simulink model "cascademodel"  (R2023a)
settings: Solver=VariableStepAuto  StartTime=0.0  StopTime=1  FixedStep=0.03  RelTol=1e-3
values from neighbouring files (symbols this model uses):
  b_1 = 51.0314    [modelsetup.m]
  b_2 = -13.8341    [modelsetup.m]
  EPSILON = 0.005    [modelsetup.m]
  F_kinetic = 8.1003    [modelsetup.m]
  F_static = 10.4160    (= 10.416)    [modelsetup.m]
  J = 9.1617    [modelsetup.m]
  K = K_t / estimated_b    (= 0.904771025438)    [modelsetup.m]
  K_t = 0.124 * 120    (= 14.88)    [modelsetup.m]
  tau = J / estimated_b    (= 0.55707262794)    [modelsetup.m]
libraries: slpidlib x5
settings Model: Creator=yunzh  LastModifiedBy=yunzh

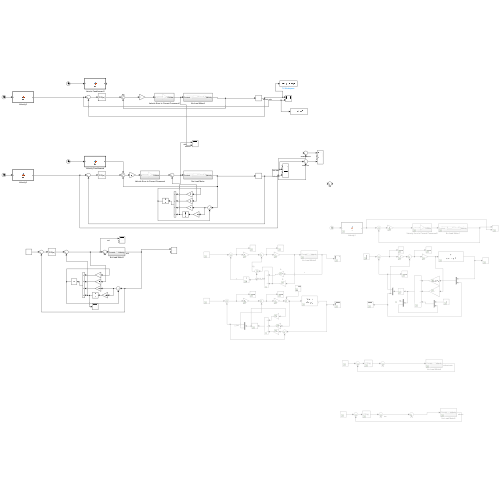
[thumbnail: Simulink's stored preview of the top-level diagram]
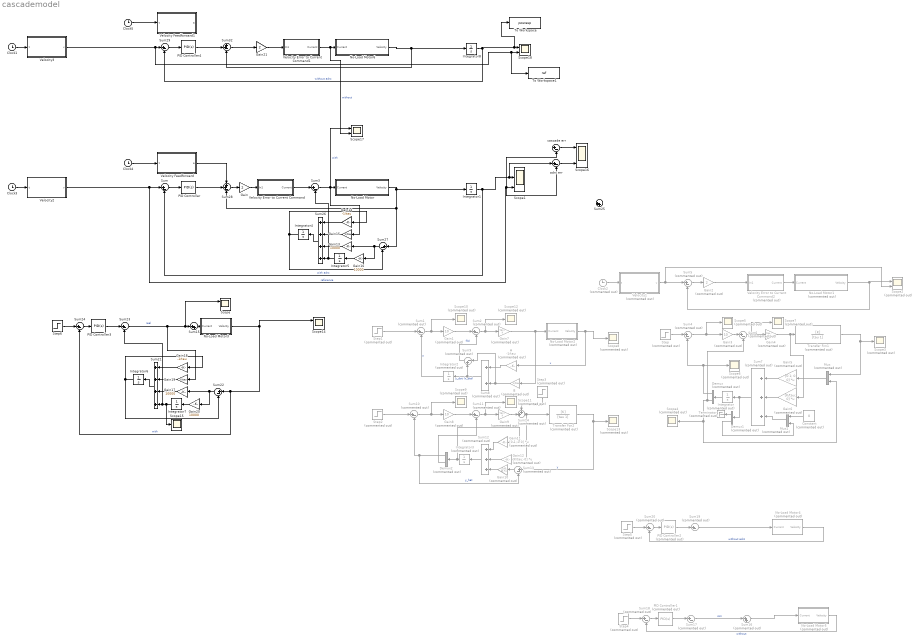
== system cascademodel ==
  A : Gain  Commented=on  Gain=-1/tau
  B : Gain  Commented=on  Gain=K/tau
  Clock{1,3..5} (4 alike) : Clock
  Clock2 : Clock  Commented=on
  Constant : Constant  Commented=on  Value=0
  Demux : Demux  Commented=on  Outputs=2
  Demux1 : Demux  Commented=on  Outputs=2
  Demux2 : Demux  Commented=on  Outputs=2
  Gain : Gain  Gain=2
  Gain1 : Gain  Commented=on  Gain=10
  Gain10 : Gain  Commented=on  Gain=[100; 0]  Multiplication=Matrix(K*u)
  Gain11 : Gain  Commented=on  Gain=[0 1; 0 0]  Multiplication=Matrix(K*u)
  Gain12 : Gain  Commented=on  Gain=[K/tau; 0]  Multiplication=Matrix(K*u)
  Gain{13,16..17,20} (4 alike) : Gain  Gain=10000
  Gain14 : Gain  Gain=-1\tau
  Gain15 : Gain  Gain=K/tau
  Gain18 : Gain  Gain=-1/tau
  Gain19 : Gain  Gain=K/tau
  Gain2 : Gain  Commented=on  Gain=2
  Gain21 : Gain  Gain=2
  Gain3 : Gain  Commented=on  Gain=10
  Gain4 : Gain  Commented=on  Gain=tau / K
  Gain5 : Gain  Commented=on  Gain=[0 1; 0 0]  Multiplication=Matrix(K*u)
  Gain6 : Gain  Commented=on  Gain=[K/tau; 0]  Multiplication=Matrix(K*u)
  Gain7 : Gain  Commented=on  Gain=tau / K
  Gain8 : Gain  Commented=on  Gain=10
  Gain9 : Gain  Commented=on  Gain=tau / K
  Integrator : Integrator  Commented=on
  Integrator{1,4..8} (6 alike) : Integrator
  Integrator2 : Integrator  Commented=on
  Integrator3 : Integrator  Commented=on
  Mux : Mux  Commented=on  Inputs=2
  Mux1 : Mux  Commented=on  Inputs=2
  No-Load Motor : Subsystem
  No-Load Motor1 : Subsystem  Commented=on
  No-Load Motor2 : Subsystem  Commented=on
  No-Load Motor3 : Subsystem
  No-Load Motor4 : Subsystem  Commented=on
  No-Load Motor5 : Subsystem  Commented=on
  No-Load Motor6 : Subsystem
  PID Controller : slpidlib/PID Controller  Controller=PID  Form=Parallel  TimeDomain=Continuous-time  UseExternalTs=off  SampleTime=-1  IntegratorMethod=Forward Euler  FilterMethod=Forward Euler  ControllerParametersSource=internal  P=10  I=1  UseKiTs=off  D=0  N=100  UseFilter=on  TunerSelectOption=Transfer Function Based (PID Tuner App)  InitialConditionSource=internal  InitialConditionForIntegrator=0  InitialConditionForFilter=0  DifferentiatorICPrevScaledInput=0  ExternalReset=none  TrackingMode=off  Kt=1  LimitOutput=off  SatLimitsSource=internal  UpperSaturationLimit=inf  LowerSaturationLimit=-inf  LinearizeAsGain=on  AntiWindupMode=none  Kb=1  LimitIntegrator=off  UpperIntegratorSaturationLimit=inf  LowerIntegratorSaturationLimit=-inf  POutMin=[]  POutMax=[]  IOutMin=[]  IOutMax=[]  DOutMin=[]  DOutMax=[]  NOutMin=[]  NOutMax=[]  SumOutMin=[]  SumOutMax=[]  SaturationOutMin=[]  SaturationOutMax=[]  PParamMin=[]  PParamMax=[]  IParamMin=[]  IParamMax=[]  DParamMin=[]  DParamMax=[]  NParamMin=[]  NParamMax=[]  KbParamMin=[]  KbParamMax=[]  KtParamMin=[]  KtParamMax=[]  KbOutMin=[]  KbOutMax=[]  KtOutMin=[]  KtOutMax=[]  IntegratorOutMin=[]  IntegratorOutMax=[]  FilterOutMin=[]  FilterOutMax=[]  SumI1OutMin=[]  SumI1OutMax=[]  SumI2OutMin=[]  SumI2OutMax=[]  SumI3OutMin=[]  SumI3OutMax=[]  SumI4OutMin=[]  SumI4OutMax=[]  SumDOutMin=[]  SumDOutMax=[]  DifferentiatorOutMin=[]  DifferentiatorOutMax=[]  FilterDiffOutCoefMin=[]  FilterDiffOutCoefMax=[]  ReciprocalOutMin=[]  ReciprocalOutMax=[]  SumDenOutMin=[]  SumDenOutMax=[]  SumNumOutMin=[]  SumNumOutMax=[]  DivideOutMin=[]  DivideOutMax=[]  UdiffTsProdOutMin=[]  UdiffTsProdOutMax=[]  NTsProdOutMin=[]  NTsProdOutMax=[]  UintegralTsProdOutMin=[]  UintegralTsProdOutMax=[]  UngainTsProdOutMin=[]  UngainTsProdOutMax=[]  ClampingZeroOutDataTypeStr=Inherit: Inherit via back propagation  ClampingZeroOutMin=[]  ClampingZeroOutMax=[]  FilterDenConstantOutDataTypeStr=Inherit: Inherit via back propagation  FilterDenConstantOutMin=[]  FilterDenConstantOutMax=[]  PCopyOutDataTypeStr=Inherit: Inherit via back propagation  PCopyOutMin=[]  PCopyOutMax=[]  NCopyOutDataTypeStr=Inherit: Inherit via back propagation  NCopyOutMin=[]  NCopyOutMax=[]  IntegratorContinuousStateAttributes=''  IntegratorStateMustResolveToSignalObject=off  IntegratorRTWStateStorageClass=Auto  FilterContinuousStateAttributes=''  FilterStateMustResolveToSignalObject=off  FilterRTWStateStorageClass=Auto  ParallelPVariant=InternalParameters  IdealPVariant=Disabled  IVariant=InternalParameters  DVariant=InternalParameters  IntegratorVariant=Continuous  SatVariant=Disabled  AWVariant=Passthrough  PCopyVariant=Disabled  TRVariant=Disabled  FdbkBlocksVariant=Forward  IdealPFdbkVariant=Disabled  SatFdbkVariant=Disabled  DerivativeFilterVariant=ContFilter  NVariant=InternalParameters  NCopyVariant=Disabled  FilterICVariant=InternalICsFilter  IntegratorICVariant=InternalICs  ExternalResetVariant=Disabled  TRSumVariant=Passthrough  SumFdbkVariant=Disabled  SumVariant=Sum_PID  TsampFilterVariant=InternalTs  TsampNgainVariant=Passthrough  TsampIntegralVariant=Disabled_SignalSpec  ExternalSaturationOutDataTypeStr=Inherit: Same as second input
  PID Controller1 : slpidlib/PID Controller  Commented=on  Controller=PID  Form=Parallel  TimeDomain=Continuous-time  UseExternalTs=off  SampleTime=-1  IntegratorMethod=Forward Euler  FilterMethod=Forward Euler  ControllerParametersSource=internal  P=5  I=1  UseKiTs=off  D=0  N=100  UseFilter=on  TunerSelectOption=Transfer Function Based (PID Tuner App)  InitialConditionSource=internal  InitialConditionForIntegrator=0  InitialConditionForFilter=0  DifferentiatorICPrevScaledInput=0  ExternalReset=none  TrackingMode=off  Kt=1  LimitOutput=off  SatLimitsSource=internal  UpperSaturationLimit=inf  LowerSaturationLimit=-inf  LinearizeAsGain=on  AntiWindupMode=none  Kb=1  LimitIntegrator=off  UpperIntegratorSaturationLimit=inf  LowerIntegratorSaturationLimit=-inf  POutMin=[]  POutMax=[]  IOutMin=[]  IOutMax=[]  DOutMin=[]  DOutMax=[]  NOutMin=[]  NOutMax=[]  SumOutMin=[]  SumOutMax=[]  SaturationOutMin=[]  SaturationOutMax=[]  PParamMin=[]  PParamMax=[]  IParamMin=[]  IParamMax=[]  DParamMin=[]  DParamMax=[]  NParamMin=[]  NParamMax=[]  KbParamMin=[]  KbParamMax=[]  KtParamMin=[]  KtParamMax=[]  KbOutMin=[]  KbOutMax=[]  KtOutMin=[]  KtOutMax=[]  IntegratorOutMin=[]  IntegratorOutMax=[]  FilterOutMin=[]  FilterOutMax=[]  SumI1OutMin=[]  SumI1OutMax=[]  SumI2OutMin=[]  SumI2OutMax=[]  SumI3OutMin=[]  SumI3OutMax=[]  SumI4OutMin=[]  SumI4OutMax=[]  SumDOutMin=[]  SumDOutMax=[]  DifferentiatorOutMin=[]  DifferentiatorOutMax=[]  FilterDiffOutCoefMin=[]  FilterDiffOutCoefMax=[]  ReciprocalOutMin=[]  ReciprocalOutMax=[]  SumDenOutMin=[]  SumDenOutMax=[]  SumNumOutMin=[]  SumNumOutMax=[]  DivideOutMin=[]  DivideOutMax=[]  UdiffTsProdOutMin=[]  UdiffTsProdOutMax=[]  NTsProdOutMin=[]  NTsProdOutMax=[]  UintegralTsProdOutMin=[]  UintegralTsProdOutMax=[]  UngainTsProdOutMin=[]  UngainTsProdOutMax=[]  ClampingZeroOutDataTypeStr=Inherit: Inherit via back propagation  ClampingZeroOutMin=[]  ClampingZeroOutMax=[]  FilterDenConstantOutDataTypeStr=Inherit: Inherit via back propagation  FilterDenConstantOutMin=[]  FilterDenConstantOutMax=[]  PCopyOutDataTypeStr=Inherit: Inherit via back propagation  PCopyOutMin=[]  PCopyOutMax=[]  NCopyOutDataTypeStr=Inherit: Inherit via back propagation  NCopyOutMin=[]  NCopyOutMax=[]  IntegratorContinuousStateAttributes=''  IntegratorStateMustResolveToSignalObject=off  IntegratorRTWStateStorageClass=Auto  FilterContinuousStateAttributes=''  FilterStateMustResolveToSignalObject=off  FilterRTWStateStorageClass=Auto  ParallelPVariant=InternalParameters  IdealPVariant=Disabled  IVariant=InternalParameters  DVariant=InternalParameters  IntegratorVariant=Continuous  SatVariant=Disabled  AWVariant=Passthrough  PCopyVariant=Disabled  TRVariant=Disabled  FdbkBlocksVariant=Forward  IdealPFdbkVariant=Disabled  SatFdbkVariant=Disabled  DerivativeFilterVariant=ContFilter  NVariant=InternalParameters  NCopyVariant=Disabled  FilterICVariant=InternalICsFilter  IntegratorICVariant=InternalICs  ExternalResetVariant=Disabled  TRSumVariant=Passthrough  SumFdbkVariant=Disabled  SumVariant=Sum_PID  TsampFilterVariant=InternalTs  TsampNgainVariant=Passthrough  TsampIntegralVariant=Disabled_SignalSpec  ExternalSaturationOutDataTypeStr=Inherit: Same as second input
  PID Controller2 : slpidlib/PID Controller  Commented=on  Controller=PID  Form=Parallel  TimeDomain=Continuous-time  UseExternalTs=off  SampleTime=-1  IntegratorMethod=Forward Euler  FilterMethod=Forward Euler  ControllerParametersSource=internal  P=1  I=1  UseKiTs=off  D=0  N=100  UseFilter=on  TunerSelectOption=Transfer Function Based (PID Tuner App)  InitialConditionSource=internal  InitialConditionForIntegrator=0  InitialConditionForFilter=0  DifferentiatorICPrevScaledInput=0  ExternalReset=none  TrackingMode=off  Kt=1  LimitOutput=off  SatLimitsSource=internal  UpperSaturationLimit=inf  LowerSaturationLimit=-inf  LinearizeAsGain=on  AntiWindupMode=none  Kb=1  LimitIntegrator=off  UpperIntegratorSaturationLimit=inf  LowerIntegratorSaturationLimit=-inf  POutMin=[]  POutMax=[]  IOutMin=[]  IOutMax=[]  DOutMin=[]  DOutMax=[]  NOutMin=[]  NOutMax=[]  SumOutMin=[]  SumOutMax=[]  SaturationOutMin=[]  SaturationOutMax=[]  PParamMin=[]  PParamMax=[]  IParamMin=[]  IParamMax=[]  DParamMin=[]  DParamMax=[]  NParamMin=[]  NParamMax=[]  KbParamMin=[]  KbParamMax=[]  KtParamMin=[]  KtParamMax=[]  KbOutMin=[]  KbOutMax=[]  KtOutMin=[]  KtOutMax=[]  IntegratorOutMin=[]  IntegratorOutMax=[]  FilterOutMin=[]  FilterOutMax=[]  SumI1OutMin=[]  SumI1OutMax=[]  SumI2OutMin=[]  SumI2OutMax=[]  SumI3OutMin=[]  SumI3OutMax=[]  SumI4OutMin=[]  SumI4OutMax=[]  SumDOutMin=[]  SumDOutMax=[]  DifferentiatorOutMin=[]  DifferentiatorOutMax=[]  FilterDiffOutCoefMin=[]  FilterDiffOutCoefMax=[]  ReciprocalOutMin=[]  ReciprocalOutMax=[]  SumDenOutMin=[]  SumDenOutMax=[]  SumNumOutMin=[]  SumNumOutMax=[]  DivideOutMin=[]  DivideOutMax=[]  UdiffTsProdOutMin=[]  UdiffTsProdOutMax=[]  NTsProdOutMin=[]  NTsProdOutMax=[]  UintegralTsProdOutMin=[]  UintegralTsProdOutMax=[]  UngainTsProdOutMin=[]  UngainTsProdOutMax=[]  ClampingZeroOutDataTypeStr=Inherit: Inherit via back propagation  ClampingZeroOutMin=[]  ClampingZeroOutMax=[]  FilterDenConstantOutDataTypeStr=Inherit: Inherit via back propagation  FilterDenConstantOutMin=[]  FilterDenConstantOutMax=[]  PCopyOutDataTypeStr=Inherit: Inherit via back propagation  PCopyOutMin=[]  PCopyOutMax=[]  NCopyOutDataTypeStr=Inherit: Inherit via back propagation  NCopyOutMin=[]  NCopyOutMax=[]  IntegratorContinuousStateAttributes=''  IntegratorStateMustResolveToSignalObject=off  IntegratorRTWStateStorageClass=Auto  FilterContinuousStateAttributes=''  FilterStateMustResolveToSignalObject=off  FilterRTWStateStorageClass=Auto  ParallelPVariant=InternalParameters  IdealPVariant=Disabled  IVariant=InternalParameters  DVariant=InternalParameters  IntegratorVariant=Continuous  SatVariant=Disabled  AWVariant=Passthrough  PCopyVariant=Disabled  TRVariant=Disabled  FdbkBlocksVariant=Forward  IdealPFdbkVariant=Disabled  SatFdbkVariant=Disabled  DerivativeFilterVariant=ContFilter  NVariant=InternalParameters  NCopyVariant=Disabled  FilterICVariant=InternalICsFilter  IntegratorICVariant=InternalICs  ExternalResetVariant=Disabled  TRSumVariant=Passthrough  SumFdbkVariant=Disabled  SumVariant=Sum_PID  TsampFilterVariant=InternalTs  TsampNgainVariant=Passthrough  TsampIntegralVariant=Disabled_SignalSpec  ExternalSaturationOutDataTypeStr=Inherit: Same as second input
  PID Controller3 : slpidlib/PID Controller  Controller=PID  Form=Parallel  TimeDomain=Continuous-time  UseExternalTs=off  SampleTime=-1  IntegratorMethod=Forward Euler  FilterMethod=Forward Euler  ControllerParametersSource=internal  P=5  I=1  UseKiTs=off  D=0  N=100  UseFilter=on  TunerSelectOption=Transfer Function Based (PID Tuner App)  InitialConditionSource=internal  InitialConditionForIntegrator=0  InitialConditionForFilter=0  DifferentiatorICPrevScaledInput=0  ExternalReset=none  TrackingMode=off  Kt=1  LimitOutput=off  SatLimitsSource=internal  UpperSaturationLimit=inf  LowerSaturationLimit=-inf  LinearizeAsGain=on  AntiWindupMode=none  Kb=1  LimitIntegrator=off  UpperIntegratorSaturationLimit=inf  LowerIntegratorSaturationLimit=-inf  POutMin=[]  POutMax=[]  IOutMin=[]  IOutMax=[]  DOutMin=[]  DOutMax=[]  NOutMin=[]  NOutMax=[]  SumOutMin=[]  SumOutMax=[]  SaturationOutMin=[]  SaturationOutMax=[]  PParamMin=[]  PParamMax=[]  IParamMin=[]  IParamMax=[]  DParamMin=[]  DParamMax=[]  NParamMin=[]  NParamMax=[]  KbParamMin=[]  KbParamMax=[]  KtParamMin=[]  KtParamMax=[]  KbOutMin=[]  KbOutMax=[]  KtOutMin=[]  KtOutMax=[]  IntegratorOutMin=[]  IntegratorOutMax=[]  FilterOutMin=[]  FilterOutMax=[]  SumI1OutMin=[]  SumI1OutMax=[]  SumI2OutMin=[]  SumI2OutMax=[]  SumI3OutMin=[]  SumI3OutMax=[]  SumI4OutMin=[]  SumI4OutMax=[]  SumDOutMin=[]  SumDOutMax=[]  DifferentiatorOutMin=[]  DifferentiatorOutMax=[]  FilterDiffOutCoefMin=[]  FilterDiffOutCoefMax=[]  ReciprocalOutMin=[]  ReciprocalOutMax=[]  SumDenOutMin=[]  SumDenOutMax=[]  SumNumOutMin=[]  SumNumOutMax=[]  DivideOutMin=[]  DivideOutMax=[]  UdiffTsProdOutMin=[]  UdiffTsProdOutMax=[]  NTsProdOutMin=[]  NTsProdOutMax=[]  UintegralTsProdOutMin=[]  UintegralTsProdOutMax=[]  UngainTsProdOutMin=[]  UngainTsProdOutMax=[]  ClampingZeroOutDataTypeStr=Inherit: Inherit via back propagation  ClampingZeroOutMin=[]  ClampingZeroOutMax=[]  FilterDenConstantOutDataTypeStr=Inherit: Inherit via back propagation  FilterDenConstantOutMin=[]  FilterDenConstantOutMax=[]  PCopyOutDataTypeStr=Inherit: Inherit via back propagation  PCopyOutMin=[]  PCopyOutMax=[]  NCopyOutDataTypeStr=Inherit: Inherit via back propagation  NCopyOutMin=[]  NCopyOutMax=[]  IntegratorContinuousStateAttributes=''  IntegratorStateMustResolveToSignalObject=off  IntegratorRTWStateStorageClass=Auto  FilterContinuousStateAttributes=''  FilterStateMustResolveToSignalObject=off  FilterRTWStateStorageClass=Auto  ParallelPVariant=InternalParameters  IdealPVariant=Disabled  IVariant=InternalParameters  DVariant=InternalParameters  IntegratorVariant=Continuous  SatVariant=Disabled  AWVariant=Passthrough  PCopyVariant=Disabled  TRVariant=Disabled  FdbkBlocksVariant=Forward  IdealPFdbkVariant=Disabled  SatFdbkVariant=Disabled  DerivativeFilterVariant=ContFilter  NVariant=InternalParameters  NCopyVariant=Disabled  FilterICVariant=InternalICsFilter  IntegratorICVariant=InternalICs  ExternalResetVariant=Disabled  TRSumVariant=Passthrough  SumFdbkVariant=Disabled  SumVariant=Sum_PID  TsampFilterVariant=InternalTs  TsampNgainVariant=Passthrough  TsampIntegralVariant=Disabled_SignalSpec  ExternalSaturationOutDataTypeStr=Inherit: Same as second input
  PID Controller4 : slpidlib/PID Controller  Controller=PID  Form=Parallel  TimeDomain=Continuous-time  UseExternalTs=off  SampleTime=-1  IntegratorMethod=Forward Euler  FilterMethod=Forward Euler  ControllerParametersSource=internal  P=10  I=1  UseKiTs=off  D=0  N=100  UseFilter=on  TunerSelectOption=Transfer Function Based (PID Tuner App)  InitialConditionSource=internal  InitialConditionForIntegrator=0  InitialConditionForFilter=0  DifferentiatorICPrevScaledInput=0  ExternalReset=none  TrackingMode=off  Kt=1  LimitOutput=off  SatLimitsSource=internal  UpperSaturationLimit=inf  LowerSaturationLimit=-inf  LinearizeAsGain=on  AntiWindupMode=none  Kb=1  LimitIntegrator=off  UpperIntegratorSaturationLimit=inf  LowerIntegratorSaturationLimit=-inf  POutMin=[]  POutMax=[]  IOutMin=[]  IOutMax=[]  DOutMin=[]  DOutMax=[]  NOutMin=[]  NOutMax=[]  SumOutMin=[]  SumOutMax=[]  SaturationOutMin=[]  SaturationOutMax=[]  PParamMin=[]  PParamMax=[]  IParamMin=[]  IParamMax=[]  DParamMin=[]  DParamMax=[]  NParamMin=[]  NParamMax=[]  KbParamMin=[]  KbParamMax=[]  KtParamMin=[]  KtParamMax=[]  KbOutMin=[]  KbOutMax=[]  KtOutMin=[]  KtOutMax=[]  IntegratorOutMin=[]  IntegratorOutMax=[]  FilterOutMin=[]  FilterOutMax=[]  SumI1OutMin=[]  SumI1OutMax=[]  SumI2OutMin=[]  SumI2OutMax=[]  SumI3OutMin=[]  SumI3OutMax=[]  SumI4OutMin=[]  SumI4OutMax=[]  SumDOutMin=[]  SumDOutMax=[]  DifferentiatorOutMin=[]  DifferentiatorOutMax=[]  FilterDiffOutCoefMin=[]  FilterDiffOutCoefMax=[]  ReciprocalOutMin=[]  ReciprocalOutMax=[]  SumDenOutMin=[]  SumDenOutMax=[]  SumNumOutMin=[]  SumNumOutMax=[]  DivideOutMin=[]  DivideOutMax=[]  UdiffTsProdOutMin=[]  UdiffTsProdOutMax=[]  NTsProdOutMin=[]  NTsProdOutMax=[]  UintegralTsProdOutMin=[]  UintegralTsProdOutMax=[]  UngainTsProdOutMin=[]  UngainTsProdOutMax=[]  ClampingZeroOutDataTypeStr=Inherit: Inherit via back propagation  ClampingZeroOutMin=[]  ClampingZeroOutMax=[]  FilterDenConstantOutDataTypeStr=Inherit: Inherit via back propagation  FilterDenConstantOutMin=[]  FilterDenConstantOutMax=[]  PCopyOutDataTypeStr=Inherit: Inherit via back propagation  PCopyOutMin=[]  PCopyOutMax=[]  NCopyOutDataTypeStr=Inherit: Inherit via back propagation  NCopyOutMin=[]  NCopyOutMax=[]  IntegratorContinuousStateAttributes=''  IntegratorStateMustResolveToSignalObject=off  IntegratorRTWStateStorageClass=Auto  FilterContinuousStateAttributes=''  FilterStateMustResolveToSignalObject=off  FilterRTWStateStorageClass=Auto  ParallelPVariant=InternalParameters  IdealPVariant=Disabled  IVariant=InternalParameters  DVariant=InternalParameters  IntegratorVariant=Continuous  SatVariant=Disabled  AWVariant=Passthrough  PCopyVariant=Disabled  TRVariant=Disabled  FdbkBlocksVariant=Forward  IdealPFdbkVariant=Disabled  SatFdbkVariant=Disabled  DerivativeFilterVariant=ContFilter  NVariant=InternalParameters  NCopyVariant=Disabled  FilterICVariant=InternalICsFilter  IntegratorICVariant=InternalICs  ExternalResetVariant=Disabled  TRSumVariant=Passthrough  SumFdbkVariant=Disabled  SumVariant=Sum_PID  TsampFilterVariant=InternalTs  TsampNgainVariant=Passthrough  TsampIntegralVariant=Disabled_SignalSpec  ExternalSaturationOutDataTypeStr=Inherit: Same as second input
  Scope{,14,17..18} (4 alike) : Scope  NumInputPorts=2
  Scope1 : Scope  NumInputPorts=4
  Scope{3..13} (11 alike) : Scope  Commented=on
  Scope15 : Scope
  Scope16 : Scope  NumInputPorts=4
  Scope2 : Scope  Commented=on  NumInputPorts=2
  Step{,1..2,4..5} (5 alike) : Step  Commented=on  SampleTime=0
  Step3 : Step  Commented=on  Time=5  After=0.2  SampleTime=0
  Step6 : Step  SampleTime=0
  Sum{,3,22..24,27,29} (7 alike) : Sum  Inputs=|+-
  Sum{1..2,4..6,10..11,13,17..20} (12 alike) : Sum  Commented=on  Inputs=|+-
  Sum12 : Sum  Commented=on  Inputs=+++
  Sum14 : Sum  Commented=on  Inputs=++|
  Sum15 : Sum  Inputs=|++
  Sum16 : Sum  Commented=on  Inputs=|++
  Sum21 : Sum  Inputs=++++
  Sum25 : Sum  Inputs=|++
  Sum26 : Sum  Inputs=++++
  Sum28 : Sum  Inputs=++-
  Sum32 : Sum  Inputs=++-
  Sum7 : Sum  Commented=on  Inputs=+++
  Sum8 : Sum  Commented=on
  Sum9 : Sum  Commented=on  Inputs=|-+
  Terminator : Terminator  Commented=on
  To Workspace : ToWorkspace  VariableName=posresp  SaveFormat=Timeseries  SampleTime=-1
  To Workspace1 : ToWorkspace  VariableName=ref  SaveFormat=Timeseries  SampleTime=-1
  Transfer Fcn1 : TransferFcn  Commented=on  Numerator=[K]  Denominator=[tau 1]
  Transfer Fcn2 : TransferFcn  Commented=on  Numerator=[K]  Denominator=[tau 1]
  Velocity Error to Current Command : Subsystem
  Velocity Error to Current Command1 : Subsystem
  Velocity Error to Current Command2 : Subsystem  Commented=on
  Velocity Feedforward : MATLAB Function  TreatAsAtomicUnit=on
  Velocity Feedforward1 : MATLAB Function  TreatAsAtomicUnit=on
  Velocity1 : MATLAB Function  Commented=on  TreatAsAtomicUnit=on
  Velocity2 : MATLAB Function  TreatAsAtomicUnit=on
  Velocity3 : MATLAB Function  TreatAsAtomicUnit=on
  adrc err : Sum  Inputs=|+-
  cascade err : Sum  Inputs=|+-
  wires:
  Sum28/1 -> Gain/1
  Gain/1 -> Velocity Error to Current Command/1(In1)
  Sum/1 -> PID Controller/1
  Integrator1/1 -> Sum/2, adrc err/1, Scope1/2  "with adrc"
  No-Load Motor/1(Velocity) -> Sum28/3, Sum27/1, Integrator1/1
  Velocity2/1(v) -> Scope1/4, adrc err/2, cascade err/2, Sum/1  "reference"
  Velocity Error to Current Command2/1(Current) -> No-Load Motor1/1(Current)
  Gain2/1 -> Velocity Error to Current Command2/1(In1)
  Sum5/1 -> Gain2/1
  No-Load Motor1/1(Velocity) -> Scope2/1, Sum5/2
  Velocity1/1(v) -> Scope2/2, Sum5/1
  Transfer Fcn1/1 -> Scope3/1, Mux/1
  Gain4/1 -> Transfer Fcn1/1, Gain6/1
  Sum4/1 -> Scope5/1, Gain3/1
  Sum6/1 -> Gain4/1, Scope7/1
  Gain3/1 -> Sum6/1
  Gain5/1 -> Sum7/1
  Gain6/1 -> Sum7/2
  Mux/1 -> Gain5/1
  Integrator/1 -> Demux/1
  Demux/2 -> Scope4/1, Mux/2, Sum6/2
  Sum7/1 -> Demux1/1, Integrator/1
  Demux/1 -> Sum4/2, Scope6/1
  Step/1 -> Sum4/1
  Clock2/1 -> Velocity1/1(t)
  Clock3/1 -> Velocity2/1(t)
  Clock4/1 -> Velocity Feedforward/1(t)
  Demux1/1 -> Terminator/1
  Demux1/2 -> Mux1/2
  Mux1/1 -> Sum7/3
  Constant/1 -> Mux1/1
  No-Load Motor2/1(Velocity) -> A/1, Scope8/1  "x"
  Gain1/1 -> Sum2/1
  Step1/1 -> Sum1/1
  Sum2/1 -> Gain7/1, Scope12/1
  Gain7/1 -> No-Load Motor2/1(Current), B/1
  Sum1/1 -> Gain1/1, Scope10/1
  B/1 -> Sum9/1, Sum8/2
  A/1 -> Sum8/1
  Sum8/1 -> Sum9/2, Integrator2/1  "y_dot (x_dot)"
  Integrator2/1 -> Sum1/2  "y"
  Sum9/1 -> Sum2/2  "f(t)"
  Gain8/1 -> Sum11/1
  Sum10/1 -> Gain8/1, Scope9/1
  Transfer Fcn2/1 -> Sum13/1, Scope13/1  "y"
  Step2/1 -> Sum10/1
  Demux2/1 -> Sum13/2, Sum10/2  "y_hat"
  Sum11/1 -> Gain9/1, Scope11/1
  Sum12/1 -> Integrator3/1
  Integrator3/1 -> Gain11/1, Demux2/1
  Demux2/2 -> Sum11/2
  Sum13/1 -> Gain10/1
  Gain10/1 -> Sum12/3
  Gain11/1 -> Sum12/1
  Gain12/1 -> Sum12/2
  Gain9/1 -> Sum14/2
  Sum14/1 -> Gain12/1, Transfer Fcn2/1
  Step3/1 -> Sum14/1
  Step4/1 -> Sum18/1
  Sum18/1 -> PID Controller1/1
  PID Controller1/1 -> Sum17/1
  Sum20/1 -> PID Controller2/1
  Step5/1 -> Sum20/1
  No-Load Motor4/1(Velocity) -> Sum20/2  "without adrc"
  Sum19/1 -> No-Load Motor4/1(Current)
  PID Controller2/1 -> Sum19/1
  No-Load Motor3/1(Velocity) -> Scope14/1, Sum24/2, Sum22/1  "with"
  Sum24/1 -> PID Controller3/1
  Integrator6/1 -> Gain18/1, Sum22/2
  Integrator7/1 -> Scope15/1, Sum23/2, Sum21/4
  Step6/1 -> Sum24/1
  Gain19/1 -> Sum21/2
  Sum21/1 -> Integrator6/1
  Gain17/1 -> Sum21/3
  Sum23/1 -> Sum15/1, Scope/1, Gain19/1  "real"
  PID Controller3/1 -> Sum23/1
  Gain18/1 -> Sum21/1
  Sum22/1 -> Gain20/1, Gain17/1
  Gain20/1 -> Integrator7/1
  No-Load Motor5/1(Velocity) -> Sum18/2  "without"
  Sum15/1 -> No-Load Motor3/1(Current)
  Sum17/1 -> Sum16/1  "sim"
  Sum16/1 -> No-Load Motor5/1(Current)
  Gain16/1 -> Integrator5/1
  Sum27/1 -> Gain16/1, Gain13/1
  Gain14/1 -> Sum26/1
  Integrator4/1 -> Gain14/1, Sum27/2
  Gain15/1 -> Sum26/2
  Integrator5/1 -> Sum3/2, Sum26/4
  Sum26/1 -> Integrator4/1
  Gain13/1 -> Sum26/3
  PID Controller/1 -> Sum28/2
  Velocity Error to Current Command/1(Current) -> Sum3/1
  Sum3/1 -> Gain15/1, No-Load Motor/1(Current), Scope17/1  "with"
  PID Controller4/1 -> Sum32/2
  Sum32/1 -> Gain21/1
  Integrator8/1 -> To Workspace/1, Scope18/1, Sum29/2  "without adrc"
  Sum29/1 -> PID Controller4/1
  Gain21/1 -> Velocity Error to Current Command1/1(In1)
  Velocity Error to Current Command1/1(Current) -> Scope17/2, No-Load Motor6/1(Current)  "without"
  Clock1/1 -> Velocity3/1(t)
  Clock5/1 -> Velocity Feedforward1/1(t)
  Velocity3/1(v) -> To Workspace1/1, Scope18/2, Sum29/1
  No-Load Motor6/1(Velocity) -> Sum32/3, Integrator8/1
  cascade err/1 -> Scope16/1
  adrc err/1 -> Scope16/4
  Velocity Feedforward/1(a) -> Sum28/1

== system cascademodel/No-Load Motor ==
  Current : Inport
  Current Torque Mapping3 : Subsystem
  Gain1 : Gain  Gain=1 / J
  Integrator : Integrator
  Velocity : Outport
  wires:
  Current Torque Mapping3/1(Output Torque) -> Gain1/1
  Gain1/1 -> Integrator/1  "Acceleration"
  Integrator/1 -> Velocity/1, Current Torque Mapping3/2(Velocity)
  Current/1 -> Current Torque Mapping3/1(Current)

== system cascademodel/No-Load Motor1 ==
  Current : Inport
  Current Torque Mapping3 : Subsystem
  Gain1 : Gain  Gain=1 / J
  Integrator : Integrator
  Velocity : Outport
  wires:
  Current Torque Mapping3/1(Output Torque) -> Gain1/1
  Gain1/1 -> Integrator/1  "Acceleration"
  Integrator/1 -> Velocity/1, Current Torque Mapping3/2(Velocity)
  Current/1 -> Current Torque Mapping3/1(Current)

== system cascademodel/No-Load Motor2 ==
  Current : Inport
  Current Torque Mapping3 : Subsystem
  Gain1 : Gain  Gain=1 / J
  Integrator : Integrator
  Velocity : Outport
  wires:
  Current Torque Mapping3/1(Output Torque) -> Gain1/1
  Gain1/1 -> Integrator/1  "Acceleration"
  Integrator/1 -> Velocity/1, Current Torque Mapping3/2(Velocity)
  Current/1 -> Current Torque Mapping3/1(Current)

== system cascademodel/No-Load Motor3 ==
  Current : Inport
  Current Torque Mapping3 : Subsystem
  Gain1 : Gain  Gain=1 / J
  Integrator : Integrator
  Velocity : Outport
  wires:
  Current Torque Mapping3/1(Output Torque) -> Gain1/1
  Gain1/1 -> Integrator/1  "Acceleration"
  Integrator/1 -> Velocity/1, Current Torque Mapping3/2(Velocity)
  Current/1 -> Current Torque Mapping3/1(Current)

== system cascademodel/No-Load Motor4 ==
  Current : Inport
  Current Torque Mapping3 : Subsystem
  Gain1 : Gain  Gain=1 / J
  Integrator : Integrator
  Velocity : Outport
  wires:
  Current Torque Mapping3/1(Output Torque) -> Gain1/1
  Gain1/1 -> Integrator/1  "Acceleration"
  Integrator/1 -> Velocity/1, Current Torque Mapping3/2(Velocity)
  Current/1 -> Current Torque Mapping3/1(Current)

== system cascademodel/No-Load Motor5 ==
  Current : Inport
  Current Torque Mapping3 : Subsystem
  Gain1 : Gain  Gain=1 / J
  Integrator : Integrator
  Velocity : Outport
  wires:
  Current Torque Mapping3/1(Output Torque) -> Gain1/1
  Gain1/1 -> Integrator/1  "Acceleration"
  Integrator/1 -> Velocity/1, Current Torque Mapping3/2(Velocity)
  Current/1 -> Current Torque Mapping3/1(Current)

== system cascademodel/No-Load Motor6 ==
  Current : Inport
  Current Torque Mapping3 : Subsystem
  Gain1 : Gain  Gain=1 / J
  Integrator : Integrator
  Velocity : Outport
  wires:
  Current Torque Mapping3/1(Output Torque) -> Gain1/1
  Gain1/1 -> Integrator/1  "Acceleration"
  Integrator/1 -> Velocity/1, Current Torque Mapping3/2(Velocity)
  Current/1 -> Current Torque Mapping3/1(Current)

== system cascademodel/Velocity Error to Current Command ==
  In1 : Inport
  Unit Conversion : Gain  Gain=180 / (pi * 3)
  Current : Outport
  wires:
  In1/1 -> Unit Conversion/1
  Unit Conversion/1 -> Current/1

== system cascademodel/Velocity Error to Current Command1 ==
  In1 : Inport
  Unit Conversion : Gain  Gain=180 / (pi * 3)
  Current : Outport
  wires:
  In1/1 -> Unit Conversion/1
  Unit Conversion/1 -> Current/1

== system cascademodel/Velocity Error to Current Command2 ==
  In1 : Inport
  Unit Conversion : Gain  Gain=180 / (pi * 3)
  Current : Outport
  wires:
  In1/1 -> Unit Conversion/1
  Unit Conversion/1 -> Current/1

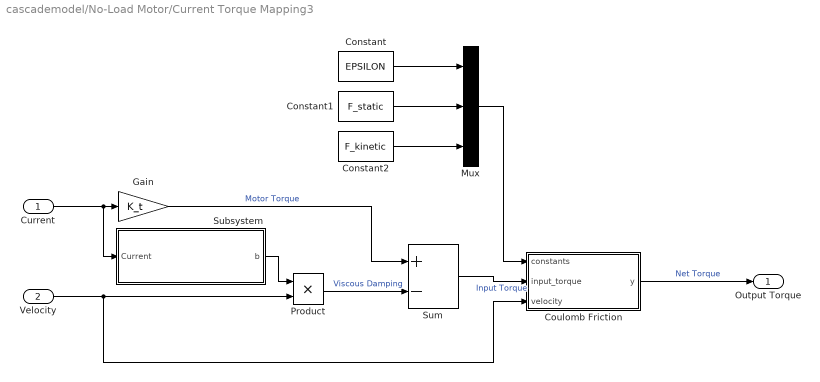
== system cascademodel/No-Load Motor/Current Torque Mapping3 ==
  Current : Inport
  Velocity : Inport  Port=2
  Constant : Constant  Value=EPSILON
  Constant1 : Constant  Value=F_static
  Constant2 : Constant  Value=F_kinetic
  Coulomb Friction : MATLAB Function  TreatAsAtomicUnit=on
  Gain : Gain  Gain=K_t
  Mux : Mux  Inputs=3
  Product : Product
  Subsystem : Subsystem
  Sum : Sum  Inputs=+-
  Output Torque : Outport
  wires:
  Constant1/1 -> Mux/2
  Gain/1 -> Sum/1  "Motor Torque"
  Mux/1 -> Coulomb Friction/1(constants)
  Sum/1 -> Coulomb Friction/2(input_torque)  "Input Torque"
  Constant/1 -> Mux/1
  Constant2/1 -> Mux/3
  Current/1 -> Subsystem/1(Current), Gain/1
  Velocity/1 -> Product/2, Coulomb Friction/3(velocity)
  Coulomb Friction/1(y) -> Output Torque/1  "Net Torque"
  Product/1 -> Sum/2  "Viscous Damping"
  Subsystem/1(b) -> Product/1

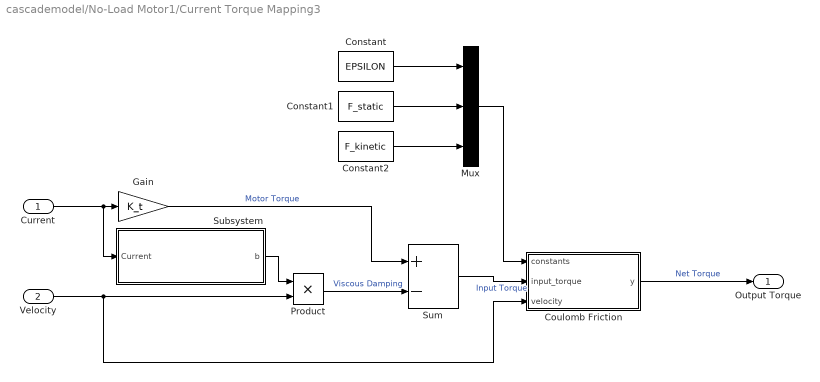
== system cascademodel/No-Load Motor1/Current Torque Mapping3 ==
  Current : Inport
  Velocity : Inport  Port=2
  Constant : Constant  Value=EPSILON
  Constant1 : Constant  Value=F_static
  Constant2 : Constant  Value=F_kinetic
  Coulomb Friction : MATLAB Function  TreatAsAtomicUnit=on
  Gain : Gain  Gain=K_t
  Mux : Mux  Inputs=3
  Product : Product
  Subsystem : Subsystem
  Sum : Sum  Inputs=+-
  Output Torque : Outport
  wires:
  Constant1/1 -> Mux/2
  Gain/1 -> Sum/1  "Motor Torque"
  Mux/1 -> Coulomb Friction/1(constants)
  Sum/1 -> Coulomb Friction/2(input_torque)  "Input Torque"
  Constant/1 -> Mux/1
  Constant2/1 -> Mux/3
  Current/1 -> Subsystem/1(Current), Gain/1
  Velocity/1 -> Product/2, Coulomb Friction/3(velocity)
  Coulomb Friction/1(y) -> Output Torque/1  "Net Torque"
  Product/1 -> Sum/2  "Viscous Damping"
  Subsystem/1(b) -> Product/1

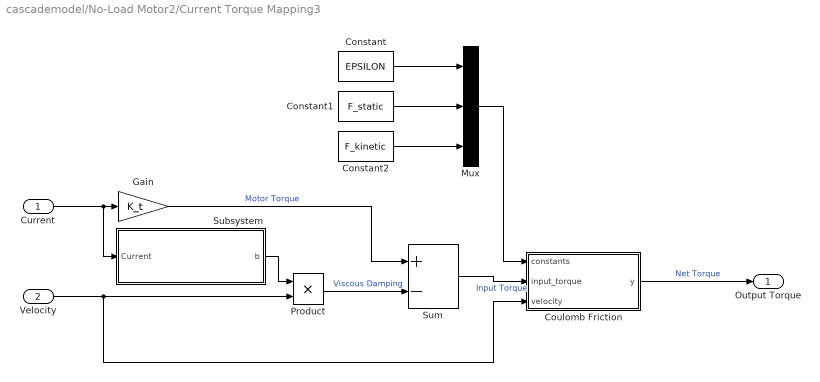
== system cascademodel/No-Load Motor2/Current Torque Mapping3 ==
  Current : Inport
  Velocity : Inport  Port=2
  Constant : Constant  Value=EPSILON
  Constant1 : Constant  Value=F_static
  Constant2 : Constant  Value=F_kinetic
  Coulomb Friction : MATLAB Function  TreatAsAtomicUnit=on
  Gain : Gain  Gain=K_t
  Mux : Mux  Inputs=3
  Product : Product
  Subsystem : Subsystem
  Sum : Sum  Inputs=+-
  Output Torque : Outport
  wires:
  Constant1/1 -> Mux/2
  Gain/1 -> Sum/1  "Motor Torque"
  Mux/1 -> Coulomb Friction/1(constants)
  Sum/1 -> Coulomb Friction/2(input_torque)  "Input Torque"
  Constant/1 -> Mux/1
  Constant2/1 -> Mux/3
  Current/1 -> Subsystem/1(Current), Gain/1
  Velocity/1 -> Product/2, Coulomb Friction/3(velocity)
  Coulomb Friction/1(y) -> Output Torque/1  "Net Torque"
  Product/1 -> Sum/2  "Viscous Damping"
  Subsystem/1(b) -> Product/1

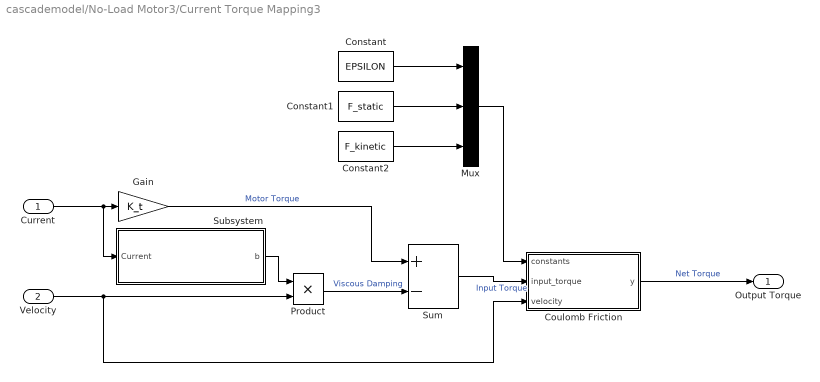
== system cascademodel/No-Load Motor3/Current Torque Mapping3 ==
  Current : Inport
  Velocity : Inport  Port=2
  Constant : Constant  Value=EPSILON
  Constant1 : Constant  Value=F_static
  Constant2 : Constant  Value=F_kinetic
  Coulomb Friction : MATLAB Function  TreatAsAtomicUnit=on
  Gain : Gain  Gain=K_t
  Mux : Mux  Inputs=3
  Product : Product
  Subsystem : Subsystem
  Sum : Sum  Inputs=+-
  Output Torque : Outport
  wires:
  Constant1/1 -> Mux/2
  Gain/1 -> Sum/1  "Motor Torque"
  Mux/1 -> Coulomb Friction/1(constants)
  Sum/1 -> Coulomb Friction/2(input_torque)  "Input Torque"
  Constant/1 -> Mux/1
  Constant2/1 -> Mux/3
  Current/1 -> Subsystem/1(Current), Gain/1
  Velocity/1 -> Product/2, Coulomb Friction/3(velocity)
  Coulomb Friction/1(y) -> Output Torque/1  "Net Torque"
  Product/1 -> Sum/2  "Viscous Damping"
  Subsystem/1(b) -> Product/1

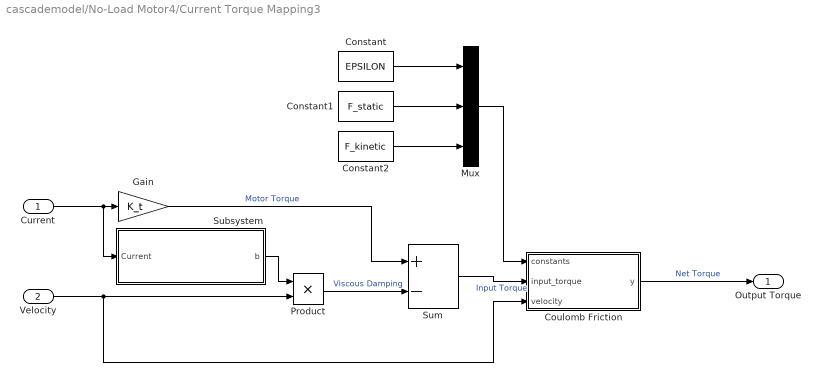
== system cascademodel/No-Load Motor4/Current Torque Mapping3 ==
  Current : Inport
  Velocity : Inport  Port=2
  Constant : Constant  Value=EPSILON
  Constant1 : Constant  Value=F_static
  Constant2 : Constant  Value=F_kinetic
  Coulomb Friction : MATLAB Function  TreatAsAtomicUnit=on
  Gain : Gain  Gain=K_t
  Mux : Mux  Inputs=3
  Product : Product
  Subsystem : Subsystem
  Sum : Sum  Inputs=+-
  Output Torque : Outport
  wires:
  Constant1/1 -> Mux/2
  Gain/1 -> Sum/1  "Motor Torque"
  Mux/1 -> Coulomb Friction/1(constants)
  Sum/1 -> Coulomb Friction/2(input_torque)  "Input Torque"
  Constant/1 -> Mux/1
  Constant2/1 -> Mux/3
  Current/1 -> Subsystem/1(Current), Gain/1
  Velocity/1 -> Product/2, Coulomb Friction/3(velocity)
  Coulomb Friction/1(y) -> Output Torque/1  "Net Torque"
  Product/1 -> Sum/2  "Viscous Damping"
  Subsystem/1(b) -> Product/1

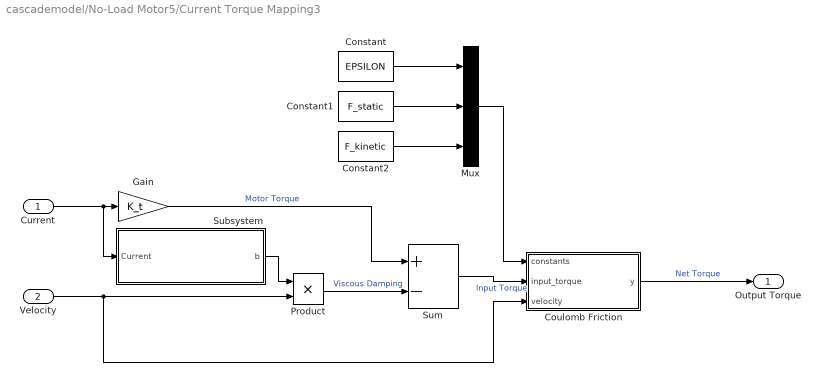
== system cascademodel/No-Load Motor5/Current Torque Mapping3 ==
  Current : Inport
  Velocity : Inport  Port=2
  Constant : Constant  Value=EPSILON
  Constant1 : Constant  Value=F_static
  Constant2 : Constant  Value=F_kinetic
  Coulomb Friction : MATLAB Function  TreatAsAtomicUnit=on
  Gain : Gain  Gain=K_t
  Mux : Mux  Inputs=3
  Product : Product
  Subsystem : Subsystem
  Sum : Sum  Inputs=+-
  Output Torque : Outport
  wires:
  Constant1/1 -> Mux/2
  Gain/1 -> Sum/1  "Motor Torque"
  Mux/1 -> Coulomb Friction/1(constants)
  Sum/1 -> Coulomb Friction/2(input_torque)  "Input Torque"
  Constant/1 -> Mux/1
  Constant2/1 -> Mux/3
  Current/1 -> Subsystem/1(Current), Gain/1
  Velocity/1 -> Product/2, Coulomb Friction/3(velocity)
  Coulomb Friction/1(y) -> Output Torque/1  "Net Torque"
  Product/1 -> Sum/2  "Viscous Damping"
  Subsystem/1(b) -> Product/1

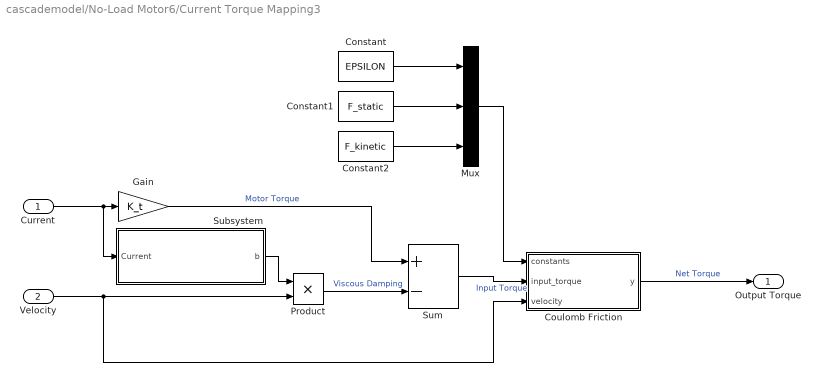
== system cascademodel/No-Load Motor6/Current Torque Mapping3 ==
  Current : Inport
  Velocity : Inport  Port=2
  Constant : Constant  Value=EPSILON
  Constant1 : Constant  Value=F_static
  Constant2 : Constant  Value=F_kinetic
  Coulomb Friction : MATLAB Function  TreatAsAtomicUnit=on
  Gain : Gain  Gain=K_t
  Mux : Mux  Inputs=3
  Product : Product
  Subsystem : Subsystem
  Sum : Sum  Inputs=+-
  Output Torque : Outport
  wires:
  Constant1/1 -> Mux/2
  Gain/1 -> Sum/1  "Motor Torque"
  Mux/1 -> Coulomb Friction/1(constants)
  Sum/1 -> Coulomb Friction/2(input_torque)  "Input Torque"
  Constant/1 -> Mux/1
  Constant2/1 -> Mux/3
  Current/1 -> Subsystem/1(Current), Gain/1
  Velocity/1 -> Product/2, Coulomb Friction/3(velocity)
  Coulomb Friction/1(y) -> Output Torque/1  "Net Torque"
  Product/1 -> Sum/2  "Viscous Damping"
  Subsystem/1(b) -> Product/1

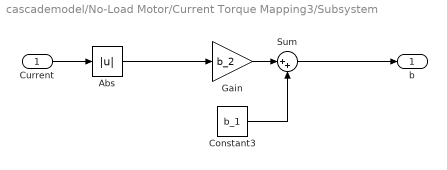
== system cascademodel/No-Load Motor/Current Torque Mapping3/Subsystem ==
  Current : Inport
  Abs : Abs  SaturateOnIntegerOverflow=off
  Constant3 : Constant  Value=b_1
  Gain : Gain  Gain=b_2
  Sum : Sum  Inputs=|++
  b : Outport
  wires:
  Current/1 -> Abs/1
  Gain/1 -> Sum/1
  Sum/1 -> b/1
  Constant3/1 -> Sum/2
  Abs/1 -> Gain/1

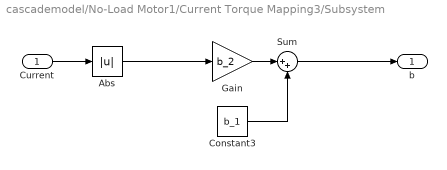
== system cascademodel/No-Load Motor1/Current Torque Mapping3/Subsystem ==
  Current : Inport
  Abs : Abs  SaturateOnIntegerOverflow=off
  Constant3 : Constant  Value=b_1
  Gain : Gain  Gain=b_2
  Sum : Sum  Inputs=|++
  b : Outport
  wires:
  Current/1 -> Abs/1
  Gain/1 -> Sum/1
  Sum/1 -> b/1
  Constant3/1 -> Sum/2
  Abs/1 -> Gain/1

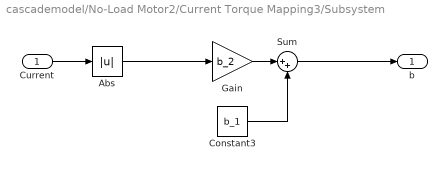
== system cascademodel/No-Load Motor2/Current Torque Mapping3/Subsystem ==
  Current : Inport
  Abs : Abs  SaturateOnIntegerOverflow=off
  Constant3 : Constant  Value=b_1
  Gain : Gain  Gain=b_2
  Sum : Sum  Inputs=|++
  b : Outport
  wires:
  Current/1 -> Abs/1
  Gain/1 -> Sum/1
  Sum/1 -> b/1
  Constant3/1 -> Sum/2
  Abs/1 -> Gain/1

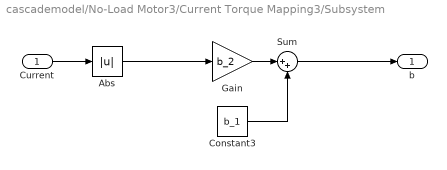
== system cascademodel/No-Load Motor3/Current Torque Mapping3/Subsystem ==
  Current : Inport
  Abs : Abs  SaturateOnIntegerOverflow=off
  Constant3 : Constant  Value=b_1
  Gain : Gain  Gain=b_2
  Sum : Sum  Inputs=|++
  b : Outport
  wires:
  Current/1 -> Abs/1
  Gain/1 -> Sum/1
  Sum/1 -> b/1
  Constant3/1 -> Sum/2
  Abs/1 -> Gain/1

== system cascademodel/No-Load Motor4/Current Torque Mapping3/Subsystem ==
  Current : Inport
  Abs : Abs  SaturateOnIntegerOverflow=off
  Constant3 : Constant  Value=b_1
  Gain : Gain  Gain=b_2
  Sum : Sum  Inputs=|++
  b : Outport
  wires:
  Current/1 -> Abs/1
  Gain/1 -> Sum/1
  Sum/1 -> b/1
  Constant3/1 -> Sum/2
  Abs/1 -> Gain/1

== system cascademodel/No-Load Motor5/Current Torque Mapping3/Subsystem ==
  Current : Inport
  Abs : Abs  SaturateOnIntegerOverflow=off
  Constant3 : Constant  Value=b_1
  Gain : Gain  Gain=b_2
  Sum : Sum  Inputs=|++
  b : Outport
  wires:
  Current/1 -> Abs/1
  Gain/1 -> Sum/1
  Sum/1 -> b/1
  Constant3/1 -> Sum/2
  Abs/1 -> Gain/1

== system cascademodel/No-Load Motor6/Current Torque Mapping3/Subsystem ==
  Current : Inport
  Abs : Abs  SaturateOnIntegerOverflow=off
  Constant3 : Constant  Value=b_1
  Gain : Gain  Gain=b_2
  Sum : Sum  Inputs=|++
  b : Outport
  wires:
  Current/1 -> Abs/1
  Gain/1 -> Sum/1
  Sum/1 -> b/1
  Constant3/1 -> Sum/2
  Abs/1 -> Gain/1

== matlab function cascademodel/Velocity3 ==
  data: t input; v output
function v = fcn(t)
    v = (3 * pi / 2) * t^2 - pi * t^3;
end

== matlab function cascademodel/No-Load Motor/Current Torque Mapping3/Coulomb Friction ==
  data: constants input; input_torque input; velocity input; y output
function y = fcn(constants, input_torque, velocity)
    EPSILON = constants(1);
    F_stat = constants(2);
    F_c = constants(3);


    if abs(velocity) < EPSILON % no motion
        if abs(input_torque) < abs(F_stat) % insufficient torque
            y = 0;
            return
        end

        % reduce torque by static friction
        static_friction = -1 * sign(input_torque) * F_stat;
        y = input_torque + static_friction;
        return
    end
    
    % reduce torque by dynamic friction
    dynamic_friction = -1 * sign(velocity) * F_c;
    y = input_torque + dynamic_friction;
end

== matlab function cascademodel/No-Load Motor2/Current Torque Mapping3/Coulomb Friction ==
  data: constants input; input_torque input; velocity input; y output
function y = fcn(constants, input_torque, velocity)
    EPSILON = constants(1);
    F_stat = constants(2);
    F_c = constants(3);


    if abs(velocity) < EPSILON % no motion
        if abs(input_torque) < abs(F_stat) % insufficient torque
            y = 0;
            return
        end

        % reduce torque by static friction
        static_friction = -1 * sign(input_torque) * F_stat;
        y = input_torque + static_friction;
        return
    end
    
    % reduce torque by dynamic friction
    dynamic_friction = -1 * sign(velocity) * F_c;
    y = input_torque + dynamic_friction;
end

== matlab function cascademodel/No-Load Motor3/Current Torque Mapping3/Coulomb Friction ==
  data: constants input; input_torque input; velocity input; y output
function y = fcn(constants, input_torque, velocity)
    EPSILON = constants(1);
    F_stat = constants(2);
    F_c = constants(3);


    if abs(velocity) < EPSILON % no motion
        if abs(input_torque) < abs(F_stat) % insufficient torque
            y = 0;
            return
        end

        % reduce torque by static friction
        static_friction = -1 * sign(input_torque) * F_stat;
        y = input_torque + static_friction;
        return
    end
    
    % reduce torque by dynamic friction
    dynamic_friction = -1 * sign(velocity) * F_c;
    y = input_torque + dynamic_friction;
end

== matlab function cascademodel/Velocity1 ==
  data: t input; v output
function v = fcn(t)
    v = (3 * pi / 200) * t^2 - pi / 1000 * t^3;
end

== matlab function cascademodel/Velocity2 ==
  data: t input; v output
function v = fcn(t)
    v = (3 * pi / 2) * t^2 - pi * t^3;
end

== matlab function cascademodel/Velocity Feedforward ==
  data: t input; a output
function a = fcn(t)
    a = (3 * pi / 2) * 2 * t - 3 * pi * t^2;
end

== matlab function cascademodel/No-Load Motor4/Current Torque Mapping3/Coulomb Friction ==
  data: constants input; input_torque input; velocity input; y output
function y = fcn(constants, input_torque, velocity)
    EPSILON = constants(1);
    F_stat = constants(2);
    F_c = constants(3);


    if abs(velocity) < EPSILON % no motion
        if abs(input_torque) < abs(F_stat) % insufficient torque
            y = 0;
            return
        end

        % reduce torque by static friction
        static_friction = -1 * sign(input_torque) * F_stat;
        y = input_torque + static_friction;
        return
    end
    
    % reduce torque by dynamic friction
    dynamic_friction = -1 * sign(velocity) * F_c;
    y = input_torque + dynamic_friction;
end

== matlab function cascademodel/No-Load Motor5/Current Torque Mapping3/Coulomb Friction ==
  data: constants input; input_torque input; velocity input; y output
function y = fcn(constants, input_torque, velocity)
    EPSILON = constants(1);
    F_stat = constants(2);
    F_c = constants(3);


    if abs(velocity) < EPSILON % no motion
        if abs(input_torque) < abs(F_stat) % insufficient torque
            y = 0;
            return
        end

        % reduce torque by static friction
        static_friction = -1 * sign(input_torque) * F_stat;
        y = input_torque + static_friction;
        return
    end
    
    % reduce torque by dynamic friction
    dynamic_friction = -1 * sign(velocity) * F_c;
    y = input_torque + dynamic_friction;
end

== matlab function cascademodel/No-Load Motor6/Current Torque Mapping3/Coulomb Friction ==
  data: constants input; input_torque input; velocity input; y output
function y = fcn(constants, input_torque, velocity)
    EPSILON = constants(1);
    F_stat = constants(2);
    F_c = constants(3);


    if abs(velocity) < EPSILON % no motion
        if abs(input_torque) < abs(F_stat) % insufficient torque
            y = 0;
            return
        end

        % reduce torque by static friction
        static_friction = -1 * sign(input_torque) * F_stat;
        y = input_torque + static_friction;
        return
    end
    
    % reduce torque by dynamic friction
    dynamic_friction = -1 * sign(velocity) * F_c;
    y = input_torque + dynamic_friction;
end

== matlab function cascademodel/No-Load Motor1/Current Torque Mapping3/Coulomb Friction ==
  data: constants input; input_torque input; velocity input; y output
function y = fcn(constants, input_torque, velocity)
    EPSILON = constants(1);
    F_stat = constants(2);
    F_c = constants(3);


    if abs(velocity) < EPSILON % no motion
        if abs(input_torque) < abs(F_stat) % insufficient torque
            y = 0;
            return
        end

        % reduce torque by static friction
        static_friction = -1 * sign(input_torque) * F_stat;
        y = input_torque + static_friction;
        return
    end
    
    % reduce torque by dynamic friction
    dynamic_friction = -1 * sign(velocity) * F_c;
    y = input_torque + dynamic_friction;
end

== matlab function cascademodel/Velocity Feedforward1 ==
  data: t input; a output
function a = fcn(t)
    a = (3 * pi / 2) * 2 * t - 3 * pi * t^2;
end
